simulink model "GyroscopeProcessing_lib_test"  (R2018b)
settings: Solver=VariableStepAuto  StartTime=0.0  StopTime=1  RelTol=1e-3
model workspace (MAT data in the model file):
  gyro_rotate_test = reshape([1 0 0 0 1 0 0 0 1 1 0 0 0 1 0 0 0 1 1 0 0 0 1 0 0 0 1], [3 3 3])
libraries: maggyroProcessing_lib x1
settings Model: Creator=Nick's PC  LastModifiedBy=Nick's PC

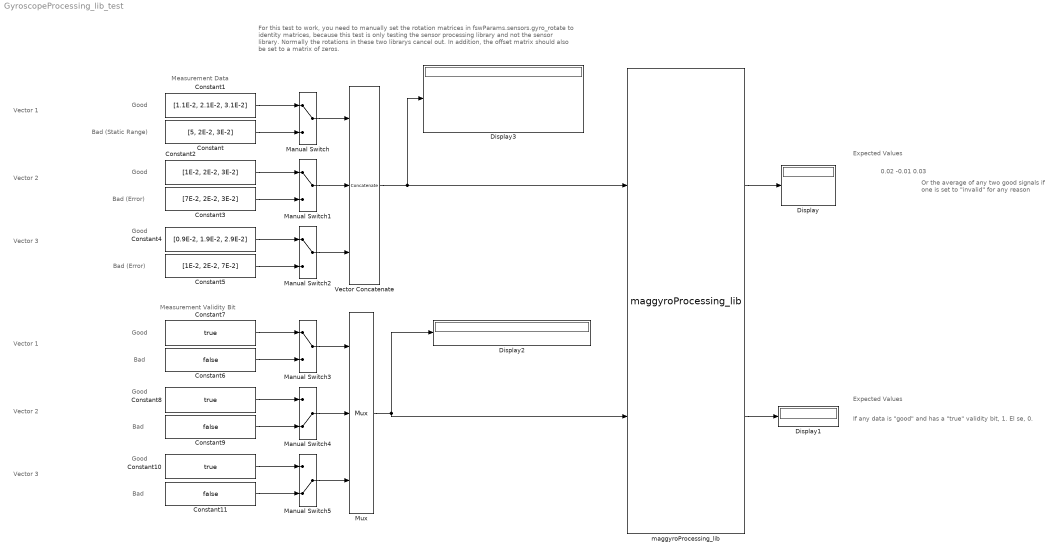
== system GyroscopeProcessing_lib_test ==
  note: For this test to work, you need to manually set the rotation matrices in fswParams.sensors.gyro_rotate to identity matrices, because
      | this test is only testing the sensor processing library and not the sensor library. Normally the rotations in these two librarys cancel out.
      | In addition, the offset matrix should also be set to a matrix of zeros.
  note: Or the average of any two good signals
      | if one is set to "invalid" for any reason
  note: Measurement Data
  note: Vector 1
  note: 0.02
      | -0.01
      | 0.03
  note: If any data is "good" and has a "true" validity bit, 1. El se, 0.
  note: Expected Values
  note: Bad (Static Range)
  note: Good
  note: Good
  note: Good
  note: Bad (Error)
  note: Bad
  note: Bad
  note: Bad
  note: Good
  note: Good
  note: Good
  note: Bad (Error)
  note: Expected Values
  note: Vector 2
  note: Vector 3
  note: Vector 2
  note: Vector 1
  note: Vector 3
  note: Measurement Validity Bit
  Constant : Constant  Value=[5, 2E-2, 3E-2]
  Constant1 : Constant  Value=[1.1E-2, 2.1E-2, 3.1E-2]
  Constant10 : Constant  Value=true
  Constant11 : Constant  Value=false
  Constant2 : Constant  Value=[1E-2, 2E-2, 3E-2]
  Constant3 : Constant  Value=[7E-2, 2E-2, 3E-2]
  Constant4 : Constant  Value=[0.9E-2, 1.9E-2, 2.9E-2]
  Constant5 : Constant  Value=[1E-2, 2E-2, 7E-2]
  Constant6 : Constant  Value=false
  Constant7 : Constant  Value=true  OutDataTypeStr=boolean
  Constant8 : Constant  Value=true
  Constant9 : Constant  Value=false
  Display{,1..3} (4 alike) : Display
  Manual Switch{,1..3} (4 alike) : ManualSwitch
  Manual Switch4 : ManualSwitch  CurrentSetting=0
  Manual Switch5 : ManualSwitch  CurrentSetting=0
  Mux : Mux  Inputs=3
  Vector Concatenate : Concatenate  NumInputs=3  Mode=Multidimensional array  ConcatenateDimension=2
  maggyroProcessing_lib : maggyroProcessing_lib/maggyroProcessing_lib  static_range_max_value=fswParams.sensors.gyro_static_range  offset_calibration_matrix=fswParams.sensors.gyro_offset  max_err=fswParams.sensors.gyro_max_err  rotation_calibration_matrix=fswParams.sensors.gyro_rotate  Gain=1
  wires:
  maggyroProcessing_lib/2 -> Display1/1
  maggyroProcessing_lib/1 -> Display/1
  Constant1/1 -> Manual Switch/1
  Constant/1 -> Manual Switch/2
  Constant2/1 -> Manual Switch1/1
  Constant3/1 -> Manual Switch1/2
  Constant4/1 -> Manual Switch2/1
  Constant5/1 -> Manual Switch2/2
  Manual Switch1/1 -> Vector Concatenate/2
  Manual Switch/1 -> Vector Concatenate/1
  Manual Switch2/1 -> Vector Concatenate/3
  Vector Concatenate/1 -> maggyroProcessing_lib/1, Display3/1
  Manual Switch5/1 -> Mux/3
  Constant10/1 -> Manual Switch5/1
  Mux/1 -> maggyroProcessing_lib/2, Display2/1
  Constant7/1 -> Manual Switch3/1
  Constant6/1 -> Manual Switch3/2
  Constant11/1 -> Manual Switch5/2
  Manual Switch4/1 -> Mux/2
  Constant8/1 -> Manual Switch4/1
  Constant9/1 -> Manual Switch4/2
  Manual Switch3/1 -> Mux/1
